simulink model "pid1"  (R2021a)
settings: Solver=VariableStepAuto  StartTime=0.0  StopTime=10.0  RelTol=1e-3
values from neighbouring files (symbols this model uses):
  c1 = 1.1*10^-7    (= 1.1e-07)    [parameter.m]
  c2 = 1.1*10^-7    (= 1.1e-07)    [parameter.m]
  c3 = 1.1*10^-7    (= 1.1e-07)    [parameter.m]
  g = 9.81    [parameter.m]
  Ix = 0.04    [parameter.m]
  Iy = 0.04    [parameter.m]
  Iz = 0.1    [parameter.m]
  k1 = 1.1*10^-7    (= 1.1e-07)    [parameter.m]
  k2 = 1.1*10^-7    (= 1.1e-07)    [parameter.m]
  k3 = 1.1*10^-7    (= 1.1e-07)    [parameter.m]
  kf = 5*10-8    (= 42)    [parameter.m]    (also in w_to_f.m = block.InputPort(5).Data)
  km = 5*10-8    (= 42)    [parameter.m]    (also in w_to_f.m = block.InputPort(6).Data)
  L = 0.25    [parameter.m]
  m = 1.535    [parameter.m]
libraries: pid_lib x4
settings Model: Creator=zlioo  LastModifiedBy=zlioo

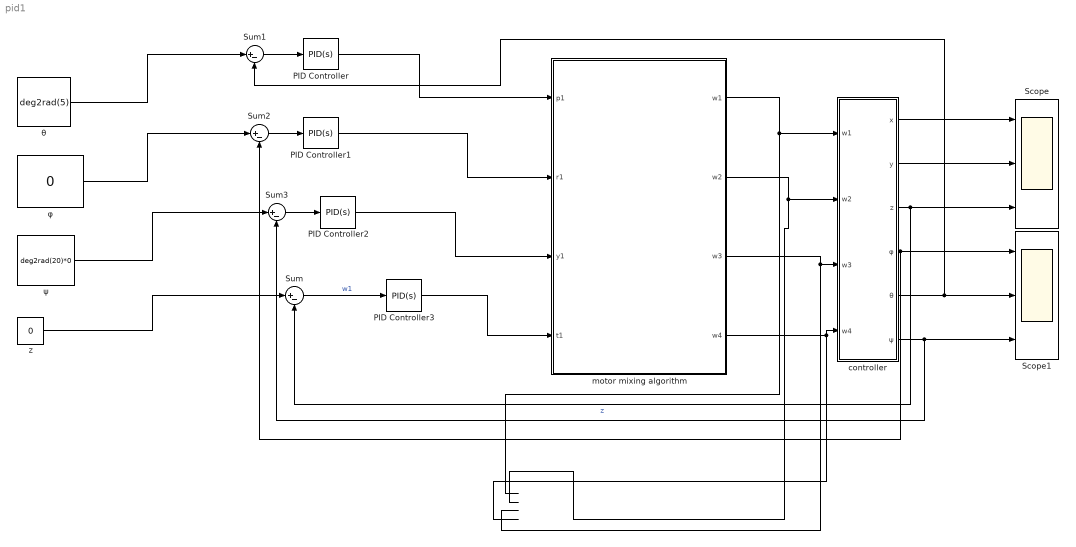
== system pid1 ==
  PID Controller : pid_lib/PID Controller  Controller=PID  Form=Parallel  TimeDomain=Continuous-time  UseExternalTs=off  SampleTime=-1  IntegratorMethod=Forward Euler  FilterMethod=Forward Euler  ControllerParametersSource=internal  P=-1.76837393576837e-05  I=-8.27860337187269e-07  D=-9.27543791921046e-05  UseFilter=on  N=5.45397025421619  TunerSelectOption=Transfer Function Based (PID Tuner App)  InitialConditionSource=internal  InitialConditionForIntegrator=0  InitialConditionForFilter=0  DifferentiatorICPrevScaledInput=0  ExternalReset=none  TrackingMode=off  Kt=1  LimitOutput=off  SatLimitsSource=internal  UpperSaturationLimit=inf  LowerSaturationLimit=-inf  LinearizeAsGain=on  AntiWindupMode=none  Kb=1  POutMin=[]  POutMax=[]  IOutMin=[]  IOutMax=[]  DOutMin=[]  DOutMax=[]  NOutMin=[]  NOutMax=[]  SumOutMin=[]  SumOutMax=[]  SaturationOutMin=[]  SaturationOutMax=[]  PParamMin=[]  PParamMax=[]  IParamMin=[]  IParamMax=[]  DParamMin=[]  DParamMax=[]  NParamMin=[]  NParamMax=[]  KbParamMin=[]  KbParamMax=[]  KtParamMin=[]  KtParamMax=[]  KbOutMin=[]  KbOutMax=[]  KtOutMin=[]  KtOutMax=[]  IntegratorOutMin=[]  IntegratorOutMax=[]  FilterOutMin=[]  FilterOutMax=[]  SumI1OutMin=[]  SumI1OutMax=[]  SumI2OutMin=[]  SumI2OutMax=[]  SumI3OutMin=[]  SumI3OutMax=[]  SumI4OutMin=[]  SumI4OutMax=[]  SumDOutMin=[]  SumDOutMax=[]  DifferentiatorOutMin=[]  DifferentiatorOutMax=[]  FilterDiffOutCoefMin=[]  FilterDiffOutCoefMax=[]  ReciprocalOutMin=[]  ReciprocalOutMax=[]  SumDenOutMin=[]  SumDenOutMax=[]  SumNumOutMin=[]  SumNumOutMax=[]  DivideOutMin=[]  DivideOutMax=[]  UdiffTsProdOutMin=[]  UdiffTsProdOutMax=[]  NTsProdOutMin=[]  NTsProdOutMax=[]  UintegralTsProdOutMin=[]  UintegralTsProdOutMax=[]  UngainTsProdOutMin=[]  UngainTsProdOutMax=[]  IntegratorContinuousStateAttributes=''  IntegratorStateMustResolveToSignalObject=off  IntegratorRTWStateStorageClass=Auto  FilterContinuousStateAttributes=''  FilterStateMustResolveToSignalObject=off  FilterRTWStateStorageClass=Auto  ParallelPVariant=InternalParameters  IdealPVariant=Disabled  IVariant=InternalParameters  DVariant=InternalParameters  IntegratorVariant=Continuous  SatVariant=Disabled  AWVariant=Passthrough  PCopyVariant=Disabled  TRVariant=Disabled  FdbkBlocksVariant=Forward  IdealPFdbkVariant=Disabled  SatFdbkVariant=Disabled  DerivativeFilterVariant=ContFilter  NVariant=InternalParameters  NCopyVariant=Disabled  FilterICVariant=InternalICsFilter  IntegratorICVariant=InternalICs  ExternalResetVariant=Disabled  TRSumVariant=Passthrough  SumFdbkVariant=Disabled  SumVariant=Sum_PID  TsampFilterVariant=InternalTs  TsampNgainVariant=Passthrough  TsampIntegralVariant=Passthrough  ExternalSaturationOutDataTypeStr=Inherit: Same as second input
  PID Controller1 : pid_lib/PID Controller  Controller=PID  Form=Parallel  TimeDomain=Continuous-time  UseExternalTs=off  SampleTime=-1  IntegratorMethod=Forward Euler  FilterMethod=Forward Euler  ControllerParametersSource=internal  P=-1.76837393592266e-05  I=-8.27860337259498e-07  D=-9.27543792001972e-05  UseFilter=on  N=5.45397025421619  TunerSelectOption=Transfer Function Based (PID Tuner App)  InitialConditionSource=internal  InitialConditionForIntegrator=0  InitialConditionForFilter=0  DifferentiatorICPrevScaledInput=0  ExternalReset=none  TrackingMode=off  Kt=1  LimitOutput=off  SatLimitsSource=internal  UpperSaturationLimit=inf  LowerSaturationLimit=-inf  LinearizeAsGain=on  AntiWindupMode=none  Kb=1  POutMin=[]  POutMax=[]  IOutMin=[]  IOutMax=[]  DOutMin=[]  DOutMax=[]  NOutMin=[]  NOutMax=[]  SumOutMin=[]  SumOutMax=[]  SaturationOutMin=[]  SaturationOutMax=[]  PParamMin=[]  PParamMax=[]  IParamMin=[]  IParamMax=[]  DParamMin=[]  DParamMax=[]  NParamMin=[]  NParamMax=[]  KbParamMin=[]  KbParamMax=[]  KtParamMin=[]  KtParamMax=[]  KbOutMin=[]  KbOutMax=[]  KtOutMin=[]  KtOutMax=[]  IntegratorOutMin=[]  IntegratorOutMax=[]  FilterOutMin=[]  FilterOutMax=[]  SumI1OutMin=[]  SumI1OutMax=[]  SumI2OutMin=[]  SumI2OutMax=[]  SumI3OutMin=[]  SumI3OutMax=[]  SumI4OutMin=[]  SumI4OutMax=[]  SumDOutMin=[]  SumDOutMax=[]  DifferentiatorOutMin=[]  DifferentiatorOutMax=[]  FilterDiffOutCoefMin=[]  FilterDiffOutCoefMax=[]  ReciprocalOutMin=[]  ReciprocalOutMax=[]  SumDenOutMin=[]  SumDenOutMax=[]  SumNumOutMin=[]  SumNumOutMax=[]  DivideOutMin=[]  DivideOutMax=[]  UdiffTsProdOutMin=[]  UdiffTsProdOutMax=[]  NTsProdOutMin=[]  NTsProdOutMax=[]  UintegralTsProdOutMin=[]  UintegralTsProdOutMax=[]  UngainTsProdOutMin=[]  UngainTsProdOutMax=[]  IntegratorContinuousStateAttributes=''  IntegratorStateMustResolveToSignalObject=off  IntegratorRTWStateStorageClass=Auto  FilterContinuousStateAttributes=''  FilterStateMustResolveToSignalObject=off  FilterRTWStateStorageClass=Auto  ParallelPVariant=InternalParameters  IdealPVariant=Disabled  IVariant=InternalParameters  DVariant=InternalParameters  IntegratorVariant=Continuous  SatVariant=Disabled  AWVariant=Passthrough  PCopyVariant=Disabled  TRVariant=Disabled  FdbkBlocksVariant=Forward  IdealPFdbkVariant=Disabled  SatFdbkVariant=Disabled  DerivativeFilterVariant=ContFilter  NVariant=InternalParameters  NCopyVariant=Disabled  FilterICVariant=InternalICsFilter  IntegratorICVariant=InternalICs  ExternalResetVariant=Disabled  TRSumVariant=Passthrough  SumFdbkVariant=Disabled  SumVariant=Sum_PID  TsampFilterVariant=InternalTs  TsampNgainVariant=Passthrough  TsampIntegralVariant=Passthrough  ExternalSaturationOutDataTypeStr=Inherit: Same as second input
  PID Controller2 : pid_lib/PID Controller  Controller=PID  Form=Parallel  TimeDomain=Continuous-time  UseExternalTs=off  SampleTime=-1  IntegratorMethod=Forward Euler  FilterMethod=Forward Euler  ControllerParametersSource=internal  P=0.000930261088313183  I=4.35499665916826e-05  D=0.00487938597079408  UseFilter=on  N=5.45397025421619  TunerSelectOption=Transfer Function Based (PID Tuner App)  InitialConditionSource=internal  InitialConditionForIntegrator=0  InitialConditionForFilter=0  DifferentiatorICPrevScaledInput=0  ExternalReset=none  TrackingMode=off  Kt=1  LimitOutput=off  SatLimitsSource=internal  UpperSaturationLimit=inf  LowerSaturationLimit=-inf  LinearizeAsGain=on  AntiWindupMode=none  Kb=1  POutMin=[]  POutMax=[]  IOutMin=[]  IOutMax=[]  DOutMin=[]  DOutMax=[]  NOutMin=[]  NOutMax=[]  SumOutMin=[]  SumOutMax=[]  SaturationOutMin=[]  SaturationOutMax=[]  PParamMin=[]  PParamMax=[]  IParamMin=[]  IParamMax=[]  DParamMin=[]  DParamMax=[]  NParamMin=[]  NParamMax=[]  KbParamMin=[]  KbParamMax=[]  KtParamMin=[]  KtParamMax=[]  KbOutMin=[]  KbOutMax=[]  KtOutMin=[]  KtOutMax=[]  IntegratorOutMin=[]  IntegratorOutMax=[]  FilterOutMin=[]  FilterOutMax=[]  SumI1OutMin=[]  SumI1OutMax=[]  SumI2OutMin=[]  SumI2OutMax=[]  SumI3OutMin=[]  SumI3OutMax=[]  SumI4OutMin=[]  SumI4OutMax=[]  SumDOutMin=[]  SumDOutMax=[]  DifferentiatorOutMin=[]  DifferentiatorOutMax=[]  FilterDiffOutCoefMin=[]  FilterDiffOutCoefMax=[]  ReciprocalOutMin=[]  ReciprocalOutMax=[]  SumDenOutMin=[]  SumDenOutMax=[]  SumNumOutMin=[]  SumNumOutMax=[]  DivideOutMin=[]  DivideOutMax=[]  UdiffTsProdOutMin=[]  UdiffTsProdOutMax=[]  NTsProdOutMin=[]  NTsProdOutMax=[]  UintegralTsProdOutMin=[]  UintegralTsProdOutMax=[]  UngainTsProdOutMin=[]  UngainTsProdOutMax=[]  IntegratorContinuousStateAttributes=''  IntegratorStateMustResolveToSignalObject=off  IntegratorRTWStateStorageClass=Auto  FilterContinuousStateAttributes=''  FilterStateMustResolveToSignalObject=off  FilterRTWStateStorageClass=Auto  ParallelPVariant=InternalParameters  IdealPVariant=Disabled  IVariant=InternalParameters  DVariant=InternalParameters  IntegratorVariant=Continuous  SatVariant=Disabled  AWVariant=Passthrough  PCopyVariant=Disabled  TRVariant=Disabled  FdbkBlocksVariant=Forward  IdealPFdbkVariant=Disabled  SatFdbkVariant=Disabled  DerivativeFilterVariant=ContFilter  NVariant=InternalParameters  NCopyVariant=Disabled  FilterICVariant=InternalICsFilter  IntegratorICVariant=InternalICs  ExternalResetVariant=Disabled  TRSumVariant=Passthrough  SumFdbkVariant=Disabled  SumVariant=Sum_PID  TsampFilterVariant=InternalTs  TsampNgainVariant=Passthrough  TsampIntegralVariant=Passthrough  ExternalSaturationOutDataTypeStr=Inherit: Same as second input
  PID Controller3 : pid_lib/PID Controller  Controller=PID  Form=Parallel  TimeDomain=Continuous-time  UseExternalTs=off  SampleTime=-1  IntegratorMethod=Forward Euler  FilterMethod=Forward Euler  ControllerParametersSource=internal  P=0.00384950942101041  I=0.000180213930030502  D=0.0201913661651451  UseFilter=on  N=5.45397025421619  TunerSelectOption=Transfer Function Based (PID Tuner App)  InitialConditionSource=internal  InitialConditionForIntegrator=0  InitialConditionForFilter=0  DifferentiatorICPrevScaledInput=0  ExternalReset=none  TrackingMode=off  Kt=1  LimitOutput=off  SatLimitsSource=internal  UpperSaturationLimit=Inf  LowerSaturationLimit=0  LinearizeAsGain=on  AntiWindupMode=none  Kb=1  POutMin=[]  POutMax=[]  IOutMin=[]  IOutMax=[]  DOutMin=[]  DOutMax=[]  NOutMin=[]  NOutMax=[]  SumOutMin=[]  SumOutMax=[]  SaturationOutMin=[]  SaturationOutMax=[]  PParamMin=[]  PParamMax=[]  IParamMin=[]  IParamMax=[]  DParamMin=[]  DParamMax=[]  NParamMin=[]  NParamMax=[]  KbParamMin=[]  KbParamMax=[]  KtParamMin=[]  KtParamMax=[]  KbOutMin=[]  KbOutMax=[]  KtOutMin=[]  KtOutMax=[]  IntegratorOutMin=[]  IntegratorOutMax=[]  FilterOutMin=[]  FilterOutMax=[]  SumI1OutMin=[]  SumI1OutMax=[]  SumI2OutMin=[]  SumI2OutMax=[]  SumI3OutMin=[]  SumI3OutMax=[]  SumI4OutMin=[]  SumI4OutMax=[]  SumDOutMin=[]  SumDOutMax=[]  DifferentiatorOutMin=[]  DifferentiatorOutMax=[]  FilterDiffOutCoefMin=[]  FilterDiffOutCoefMax=[]  ReciprocalOutMin=[]  ReciprocalOutMax=[]  SumDenOutMin=[]  SumDenOutMax=[]  SumNumOutMin=[]  SumNumOutMax=[]  DivideOutMin=[]  DivideOutMax=[]  UdiffTsProdOutMin=[]  UdiffTsProdOutMax=[]  NTsProdOutMin=[]  NTsProdOutMax=[]  UintegralTsProdOutMin=[]  UintegralTsProdOutMax=[]  UngainTsProdOutMin=[]  UngainTsProdOutMax=[]  IntegratorContinuousStateAttributes=''  IntegratorStateMustResolveToSignalObject=off  IntegratorRTWStateStorageClass=Auto  FilterContinuousStateAttributes=''  FilterStateMustResolveToSignalObject=off  FilterRTWStateStorageClass=Auto  ParallelPVariant=InternalParameters  IdealPVariant=Disabled  IVariant=InternalParameters  DVariant=InternalParameters  IntegratorVariant=Continuous  SatVariant=Disabled  AWVariant=Passthrough  PCopyVariant=Disabled  TRVariant=Disabled  FdbkBlocksVariant=Forward  IdealPFdbkVariant=Disabled  SatFdbkVariant=Disabled  DerivativeFilterVariant=ContFilter  NVariant=InternalParameters  NCopyVariant=Disabled  FilterICVariant=InternalICsFilter  IntegratorICVariant=InternalICs  ExternalResetVariant=Disabled  TRSumVariant=Passthrough  SumFdbkVariant=Disabled  SumVariant=Sum_PID  TsampFilterVariant=InternalTs  TsampNgainVariant=Passthrough  TsampIntegralVariant=Passthrough  ExternalSaturationOutDataTypeStr=Inherit: Same as second input
  Scope : Scope  NumInputPorts=3
  Scope1 : Scope  NumInputPorts=3
  Sum{,1..3} (4 alike) : Sum  Inputs=|+-
  controller : Subsystem
  motor mixing algorithm : Subsystem
  z : Constant  Value=0
  θ : Constant  Value=deg2rad(5)
  φ : Constant  Value=0
  ψ : Constant  Value=deg2rad(20)*0
  wires:
  PID Controller3/1 -> motor mixing algorithm/4(t1)
  Sum2/1 -> PID Controller1/1
  Sum/1 -> PID Controller3/1  "w1"
  motor mixing algorithm/1(w1) -> controller/1(w1)
  motor mixing algorithm/3(w3) -> controller/3(w3)
  motor mixing algorithm/4(w4) -> controller/4(w4)
  PID Controller2/1 -> motor mixing algorithm/3(y1)
  φ/1 -> Sum2/1
  Sum3/1 -> PID Controller2/1
  ψ/1 -> Sum3/1
  θ/1 -> Sum1/1
  Sum1/1 -> PID Controller/1
  controller/5(θ) -> Scope1/2, Sum1/2
  controller/6(ψ) -> Sum3/2, Scope1/3
  motor mixing algorithm/2(w2) -> controller/2(w2)
  controller/2(y) -> Scope/2
  PID Controller1/1 -> motor mixing algorithm/2(r1)
  controller/1(x) -> Scope/1
  PID Controller/1 -> motor mixing algorithm/1(p1)
  controller/3(z) -> Scope/3, Sum/2  "z"
  z/1 -> Sum/1
  controller/4(φ) -> Scope1/1, Sum2/2

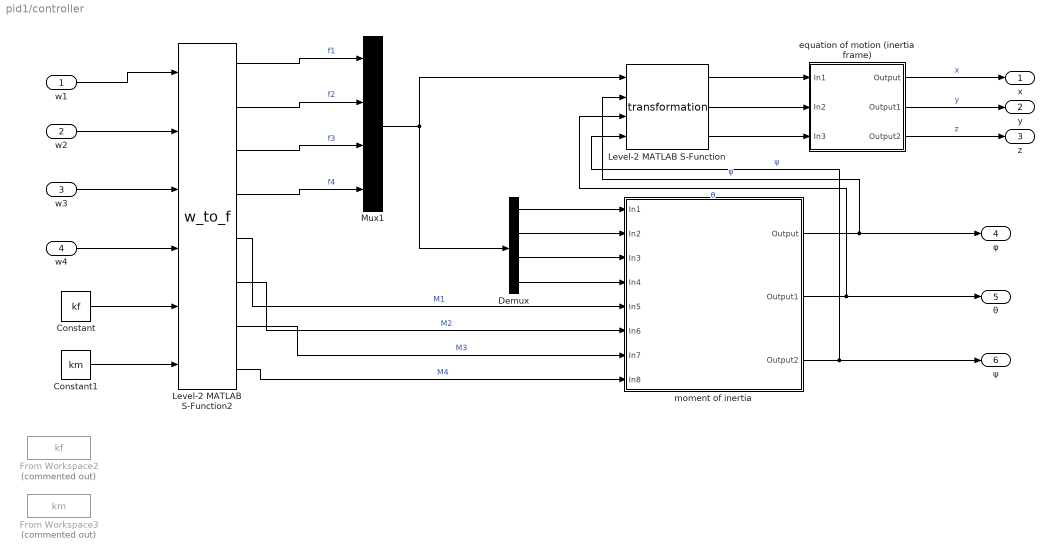
== system pid1/controller ==
  w1 : Inport
  w2 : Inport  Port=2
  w3 : Inport  Port=3
  w4 : Inport  Port=4
  Constant : Constant  Value=kf
  Constant1 : Constant  Value=km
  Demux : Demux
  From Workspace2 : FromWorkspace  Commented=on  VariableName=kf
  From Workspace3 : FromWorkspace  Commented=on  VariableName=km
  Level-2 MATLAB S-Function : M-S-Function  FunctionName=transformation
  Level-2 MATLAB S-Function2 : M-S-Function  FunctionName=w_to_f
  Mux1 : Mux
  equation of motion (inertia frame) : Subsystem
  moment of inertia : Subsystem
  x : Outport
  y : Outport  Port=2
  z : Outport  Port=3
  φ : Outport  Port=4
  θ : Outport  Port=5
  ψ : Outport  Port=6
  wires:
  Level-2 MATLAB S-Function2/4 -> Mux1/4  "f4"
  Level-2 MATLAB S-Function/3 -> equation of motion (inertia frame)/3(In3)
  Demux/3 -> moment of inertia/3(In3)
  moment of inertia/3(Output2) -> ψ/1, Level-2 MATLAB S-Function/4  "ψ"
  Level-2 MATLAB S-Function2/5 -> moment of inertia/5(In5)  "M1"
  moment of inertia/2(Output1) -> θ/1, Level-2 MATLAB S-Function/3  "θ"
  equation of motion (inertia frame)/2(Output1) -> y/1  "y"
  Level-2 MATLAB S-Function2/6 -> moment of inertia/6(In6)  "M2"
  Level-2 MATLAB S-Function/1 -> equation of motion (inertia frame)/1(In1)
  Demux/1 -> moment of inertia/1(In1)
  moment of inertia/1(Output) -> φ/1, Level-2 MATLAB S-Function/2  "φ"
  w3/1 -> Level-2 MATLAB S-Function2/3
  Demux/4 -> moment of inertia/4(In4)
  Demux/2 -> moment of inertia/2(In2)
  Level-2 MATLAB S-Function2/1 -> Mux1/1  "f1"
  Level-2 MATLAB S-Function2/3 -> Mux1/3  "f3"
  Level-2 MATLAB S-Function2/7 -> moment of inertia/7(In7)  "M3"
  Level-2 MATLAB S-Function2/8 -> moment of inertia/8(In8)  "M4"
  Level-2 MATLAB S-Function2/2 -> Mux1/2  "f2"
  Mux1/1 -> Level-2 MATLAB S-Function/1, Demux/1
  w1/1 -> Level-2 MATLAB S-Function2/1
  Level-2 MATLAB S-Function/2 -> equation of motion (inertia frame)/2(In2)
  equation of motion (inertia frame)/3(Output2) -> z/1  "z"
  w4/1 -> Level-2 MATLAB S-Function2/4
  equation of motion (inertia frame)/1(Output) -> x/1  "x"
  w2/1 -> Level-2 MATLAB S-Function2/2
  Constant/1 -> Level-2 MATLAB S-Function2/5
  Constant1/1 -> Level-2 MATLAB S-Function2/6

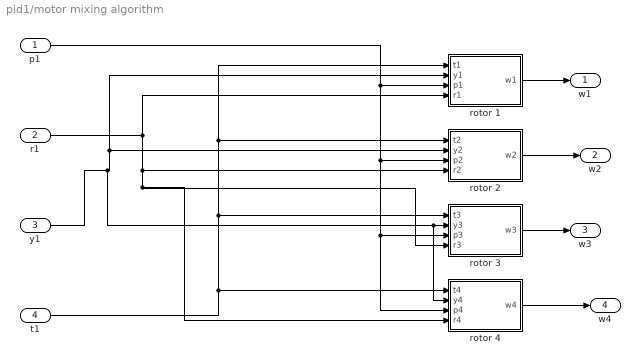
== system pid1/motor mixing algorithm ==
  p1 : Inport
  r1 : Inport  Port=2
  y1 : Inport  Port=3
  t1 : Inport  Port=4
  rotor 1 : MATLAB Function  TreatAsAtomicUnit=on
  rotor 2 : MATLAB Function  TreatAsAtomicUnit=on
  rotor 3 : MATLAB Function  TreatAsAtomicUnit=on
  rotor 4 : MATLAB Function  TreatAsAtomicUnit=on
  w1 : Outport
  w2 : Outport  Port=2
  w3 : Outport  Port=3
  w4 : Outport  Port=4
  wires:
  t1/1 -> rotor 3/1(t3), rotor 2/1(t2), rotor 1/1(t1), rotor 4/1(t4)
  rotor 1/1(w1) -> w1/1
  y1/1 -> rotor 4/2(y4), rotor 3/2(y3), rotor 2/2(y2), rotor 1/2(y1)
  r1/1 -> rotor 1/4(r1), rotor 4/4(r4), rotor 3/4(r3), rotor 2/4(r2)
  rotor 3/1(w3) -> w3/1
  p1/1 -> rotor 4/3(p4), rotor 3/3(p3), rotor 2/3(p2), rotor 1/3(p1)
  rotor 2/1(w2) -> w2/1
  rotor 4/1(w4) -> w4/1

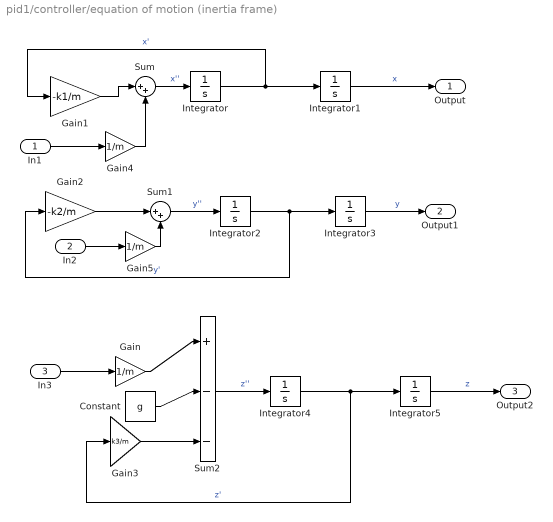
== system pid1/controller/equation of motion (inertia frame) ==
  In1 : Inport
  In2 : Inport  Port=2
  In3 : Inport  Port=3
  Constant : Constant  Value=g
  Gain : Gain  Gain=1/m
  Gain1 : Gain  Gain=-k1/m
  Gain2 : Gain  Gain=-k2/m
  Gain3 : Gain  Gain=k3/m
  Gain4 : Gain  Gain=1/m
  Gain5 : Gain  Gain=1/m
  Integrator{,1..5} (6 alike) : Integrator
  Sum : Sum  Inputs=|++
  Sum1 : Sum  Inputs=|++
  Sum2 : Sum  Inputs=|+--
  Output : Outport
  Output1 : Outport  Port=2
  Output2 : Outport  Port=3
  wires:
  Integrator/1 -> Gain1/1, Integrator1/1  "x'"
  Integrator2/1 -> Gain2/1, Integrator3/1  "y'"
  Integrator4/1 -> Integrator5/1, Gain3/1  "z'"
  Sum/1 -> Integrator/1  "x''"
  Gain1/1 -> Sum/1
  Gain2/1 -> Sum1/1
  Sum1/1 -> Integrator2/1  "y''"
  Integrator1/1 -> Output/1  "x"
  Integrator3/1 -> Output1/1  "y"
  Integrator5/1 -> Output2/1  "z"
  In3/1 -> Gain/1
  Gain/1 -> Sum2/1
  Constant/1 -> Sum2/2
  Gain3/1 -> Sum2/3
  Sum2/1 -> Integrator4/1  "z''"
  In1/1 -> Gain4/1
  Gain4/1 -> Sum/2
  In2/1 -> Gain5/1
  Gain5/1 -> Sum1/2

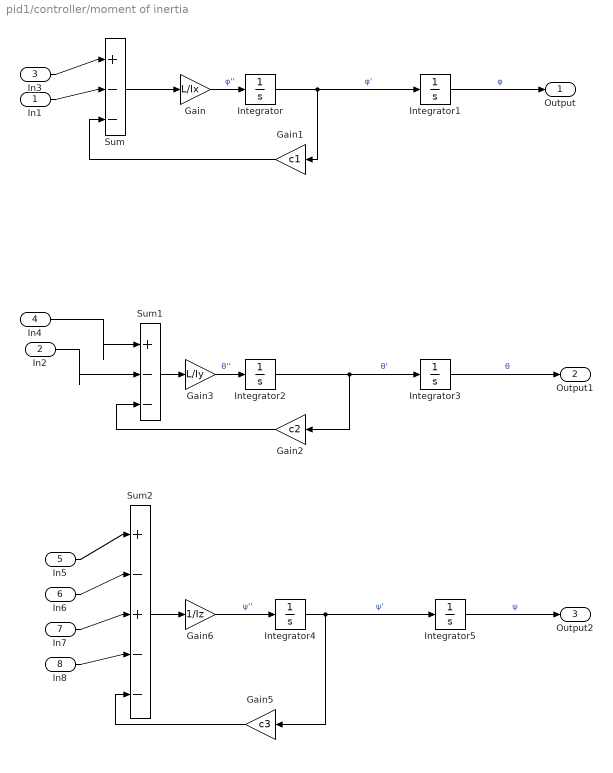
== system pid1/controller/moment of inertia ==
  In1 : Inport
  In2 : Inport  Port=2
  In3 : Inport  Port=3
  In4 : Inport  Port=4
  In5 : Inport  Port=5
  In6 : Inport  Port=6
  In7 : Inport  Port=7
  In8 : Inport  Port=8
  Gain : Gain  Gain=L/Ix
  Gain1 : Gain  Gain=c1
  Gain2 : Gain  Gain=c2
  Gain3 : Gain  Gain=L/Iy
  Gain5 : Gain  Gain=c3
  Gain6 : Gain  Gain=1/Iz
  Integrator{,1..5} (6 alike) : Integrator
  Sum : Sum  Inputs=|+--
  Sum1 : Sum  Inputs=|+--
  Sum2 : Sum  Inputs=|+-+--
  Output : Outport
  Output1 : Outport  Port=2
  Output2 : Outport  Port=3
  wires:
  Integrator/1 -> Gain1/1, Integrator1/1  "φ'"
  Integrator2/1 -> Gain2/1, Integrator3/1  "θ'"
  Integrator4/1 -> Gain5/1, Integrator5/1  "ψ'"
  Integrator1/1 -> Output/1  "φ"
  Integrator3/1 -> Output1/1  "θ"
  Integrator5/1 -> Output2/1  "ψ"
  Gain6/1 -> Integrator4/1  "ψ''"
  In3/1 -> Sum/1
  In1/1 -> Sum/2
  Gain1/1 -> Sum/3
  Sum/1 -> Gain/1
  Gain/1 -> Integrator/1  "φ''"
  Gain2/1 -> Sum1/3
  In2/1 -> Sum1/2
  In4/1 -> Sum1/1
  Sum1/1 -> Gain3/1
  Gain3/1 -> Integrator2/1  "θ''"
  In7/1 -> Sum2/3
  In8/1 -> Sum2/4
  Gain5/1 -> Sum2/5
  Sum2/1 -> Gain6/1
  In6/1 -> Sum2/2
  In5/1 -> Sum2/1

== matlab function pid1/motor mixing algorithm/rotor 1 ==
  data: t1 input; w1 output; y1 input; p1 input; r1 input
function w1 = fcn(t1,y1,p1,r1)

w1 = t1-y1-p1+0;

== matlab function pid1/motor mixing algorithm/rotor 2 ==
  data: t2 input; w2 output; y2 input; p2 input; r2 input
function w2 = fcn(t2,y2,p2,r2)

w2 = t2+y2+0+r2;

== matlab function pid1/motor mixing algorithm/rotor 3 ==
  data: t3 input; w3 output; y3 input; p3 input; r3 input
function w3 = fcn(t3,y3,p3,r3)

w3 = t3-y3+p3+0;

== matlab function pid1/motor mixing algorithm/rotor 4 ==
  data: t4 input; w4 output; y4 input; p4 input; r4 input
function w4 = fcn(t4,y4,p4,r4)

w4 = t4+y4+0-r4;
